simulink model "MomentumBasedController"  (R2021b)
settings: Solver=FixedStepAuto  StartTime=0.0  StopTime=Config.SIMULATION_TIME  FixedStep=Config.tStep  RelTol=1e-3
InitFcn:
  | %% initialize the simulation
  | cd(fileparts(which(bdroot)));
  | initMomentumBasedController;
StopFcn:
  | %% stop the simulation
  | cd(fileparts(which(bdroot)));
  | stopMomentumBasedController;
values from neighbouring files (symbols this model uses):
  ConfigRobot1 = ConfigRobot    [initMomentumBasedController.m]
undefined symbols (not defined in the file or in its folder): Config
libraries: RobotStateLibrary x16, WBToolboxLibrary x14, simulink x2
settings Model: Creator=lorenzorapetti  LastModifiedBy=lorenzorapetti
settings SolverCC: AlgebraicLoopSolver=TrustRegion
settings DebuggingCC: SFMachineParentedDataDiag=warning

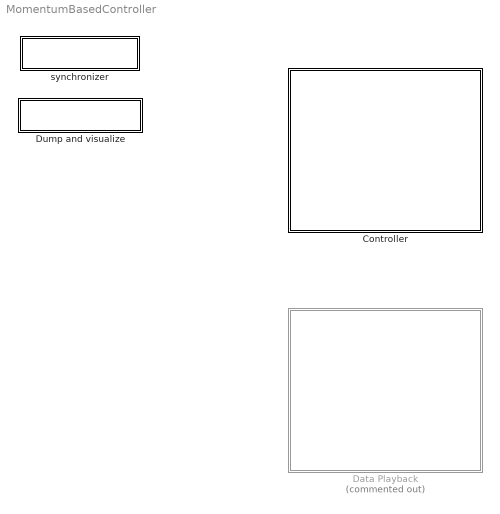
== system MomentumBasedController ==
  Controller : Subsystem
  Data Playback : Subsystem  Commented=on
  Dump and visualize : Subsystem
      mask Display: disp('VISUALIZER')
  synchronizer : Subsystem
      mask Display: disp('SYNCHRONIZER')

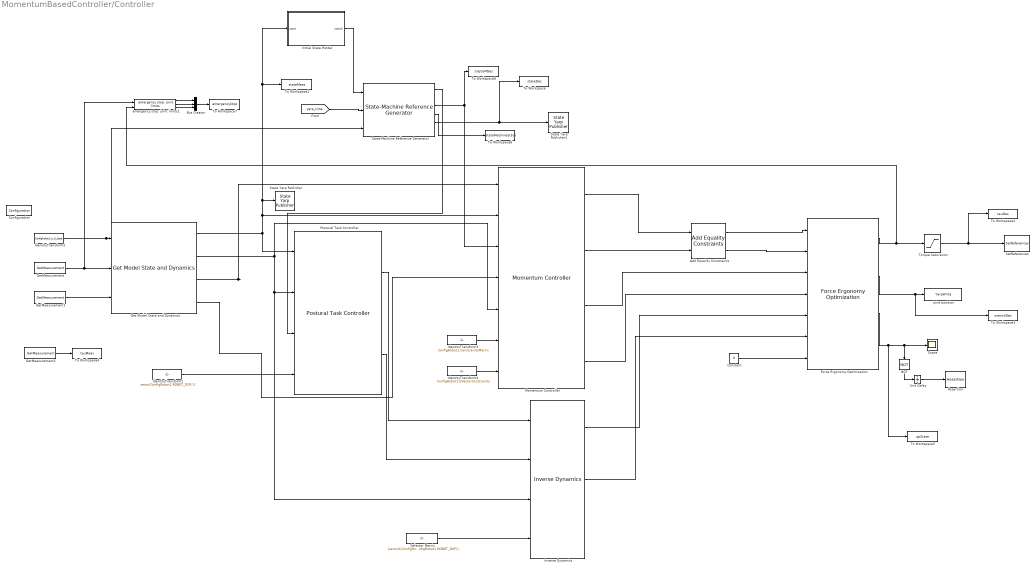
== system MomentumBasedController/Controller ==
  Add Equality Constraints : RobotStateLibrary/Add Equality Constraints  Aeq_add=ConfigRobot1.wrench_Aeq_const  beq_add=ConfigRobot1.wrench_beq_const
      settings: SourceProductName=robot-state-library
  Assertion : Assertion
  Bus Creator : BusCreator  Inputs=3
  Configuration : WBToolboxLibrary/Utilities/Configuration  ConfigSource=Workspace  ConfigObject='WBTConfigRobot_1'
      settings: SourceProductName=WholeBodyToolbox
  Constant : Constant  Value=0
  Force Ergonomy Optimization : RobotStateLibrary/Force Ergonomy Optimization  InvTol=ConfigRobot1.Reg.AInvTol  regularizationHessian=ConfigRobot1.Reg.Hessian  minimizationWeight=ConfigRobot1.Gains.tauMinimization  regularizationYDes=0
      settings: SourceProductName=robot-state-library
  Get Model State and Dynamics : RobotStateLibrary/Get Model State and Dynamics  nDoF=ConfigRobot1.ROBOT_DOF  regularization=0.001  contactFrame1Name=ConfigRobot1.Frames.LEFT_FOOT  contactFrame2Name=ConfigRobot1.Frames.RIGHT_FOOT  frame1=ConfigRobot1.Frames.LEFT_FOOT  frame2=ConfigRobot1.Frames.RIGHT_FOOT  frame3=ConfigRobot1.Frames.LEFT_HAND  frame4=ConfigRobot1.Frames.RIGHT_HAND
      settings: SourceProductName=robot-state-library
  GetMeasurement : WBToolboxLibrary/States/GetMeasurement  measuredType=Joints Position
      settings: SourceProductName=WholeBodyToolbox
  GetMeasurement1 : WBToolboxLibrary/States/GetMeasurement  measuredType=Joints Velocity
      settings: SourceProductName=WholeBodyToolbox
  GetMeasurement2 : WBToolboxLibrary/States/GetMeasurement  measuredType=Joints Torque
      settings: SourceProductName=WholeBodyToolbox
  IdentityTransform1 : Constant  Value=zeros(ConfigRobot1.ROBOT_DOF,1)
  IdentityTransform2 : Constant  Value=ConfigRobot1.w_H_base
  IdentityTransform3 : Constant  Value=ConfigRobot1.ConstraintsMatrix
  IdentityTransform4 : Constant  Value=ConfigRobot1.bVectorConstraints
  Initial State Holder : Subsystem
  Inverse Dynamics : RobotStateLibrary/Inverse Dynamics  Reg=ConfigRobot1.Reg  fixedLinkVelcityComponents=ConfigRobot1.fixedLinkVelcityComponents
      settings: SourceProductName=robot-state-library
  Momentum Controller : RobotStateLibrary/Momentum Controller  GainMomentum=ConfigRobot1.Gains.GainMomentum  linksUseConstraintMatrix=ConfigRobot1.linksUseConstraintMatrix
      settings: SourceProductName=robot-state-library
  NOT : Logic  Operator=NOT  IconShape=distinctive  AllPortsSameDT=off  OutDataTypeStr=boolean
  Postural Task Controller : RobotStateLibrary/Postural Task Controller  GainPostural=ConfigRobot1.Gains.GainPostural
      settings: SourceProductName=robot-state-library
  Scope : Scope
  Selector Matrix : Constant  Value=[zeros(6,ConfigRobot1.ROBOT_DOF); eye(ConfigRobot1.ROBOT_DOF)]
  SetReferences : WBToolboxLibrary/Actuators/SetReferences  controlType=Torque  refSpeed=10*(pi/180)  refAcceleration=1000000*(pi/180)
      settings: SourceProductName=WholeBodyToolbox
  State Yarp Publisher : RobotStateLibrary/State Yarp Publisher  basePosePortName='/collaborativeController/robot1/basePose:o'  jointPosPortName='/collaborativeController/robot1/jointPosition:o'  nuPortName='/collaborativeController/robot1/stateVelocity:o'  posCoMPortName='/collaborativeController/robot1/CoMPosition:o'
      settings: SourceProductName=robot-state-library
  State Yarp Publisher1 : RobotStateLibrary/State Yarp Publisher  basePosePortName='/collaborativeController/robotRef/basePose:o'  jointPosPortName='/collaborativeController/robotRef/jointPosition:o'  nuPortName='/collaborativeController/robotRef/stateVelocity:o'  posCoMPortName='/collaborativeController/robotRef/CoMPosition:o'
      settings: SourceProductName=robot-state-library
  State-Machine Reference Generator : RobotStateLibrary/State-Machine Reference Generator  configStateMachine=ConfigRobot1.StateMachine  sampleTime=Config.tStep  frameName1=ConfigRobot1.Frames.LEFT_FOOT  frameName2=ConfigRobot1.Frames.RIGHT_FOOT  regularization=0.001  nDoF=ConfigRobot1.ROBOT_DOF  frame1=ConfigRobot1.Frames.LEFT_FOOT  frame2=ConfigRobot1.Frames.RIGHT_FOOT  frame3=ConfigRobot1.Frames.LEFT_HAND  frame4=ConfigRobot1.Frames.RIGHT_HAND
      link override "CoM6D ->  CoMXYZ2": NumberOfDimensions=1  InputPortWidth=6
      link override "CoM6D ->  CoMXYZ5": NumberOfDimensions=1  InputPortWidth=-1
      settings: SourceProductName=robot-state-library
  To Workspace : ToWorkspace  VariableName=stateDes  SaveFormat=Timeseries  SampleTime=-1
  To Workspace1 : ToWorkspace  VariableName=stateMeas  SaveFormat=Timeseries  SampleTime=-1
  To Workspace2 : ToWorkspace  VariableName=tauDes  SaveFormat=Timeseries  SampleTime=-1
  To Workspace3 : ToWorkspace  VariableName=wrenchDes  SaveFormat=Timeseries  SampleTime=-1
  To Workspace4 : ToWorkspace  VariableName=tauMeas  SaveFormat=Timeseries  SampleTime=-1
  To Workspace5 : ToWorkspace  VariableName=qpState  SaveFormat=Timeseries  SampleTime=-1
  To Workspace6 : ToWorkspace  VariableName=stateMachineState  SaveFormat=Timeseries  SampleTime=-1
  To Workspace7 : ToWorkspace  VariableName=emergencyStop  SaveFormat=Timeseries  SampleTime=-1
  To Workspace8 : ToWorkspace  VariableName=trajCoMDes  SaveFormat=Timeseries  SampleTime=-1
  Torque Saturation : Saturate  UpperLimit=ConfigRobot1.Safety.torqueSaturation  LowerLimit=-ConfigRobot1.Safety.torqueSaturation
  Unit Delay : UnitDelay  InitialCondition=1  SampleTime=Config.tStep  HasFrameUpgradeWarning=on
  emergency stop: joint limits1 : RobotStateLibrary/emergency stop: joint limits  Safety=ConfigRobot1.Safety
      settings: SourceProductName=robot-state-library
  joint position : WBToolboxLibrary/Utilities/YarpWrite  portName='/collaborativeController/robotRef/wrench:o'  autoconnect=off  errorOnConnection=on
      settings: SourceProductName=WholeBodyToolbox
  wires:
  IdentityTransform1/1 -> Postural Task Controller/4
  GetMeasurement/1 -> emergency stop: joint limits1/1, Get Model State and Dynamics/2
  GetMeasurement1/1 -> Get Model State and Dynamics/3
  IdentityTransform2/1 -> State-Machine Reference Generator/3, Get Model State and Dynamics/1
  Get Model State and Dynamics/3 -> Momentum Controller/1
  State-Machine Reference Generator/3 -> Momentum Controller/3, To Workspace8/1
  IdentityTransform3/1 -> Momentum Controller/6
  IdentityTransform4/1 -> Momentum Controller/7
  Postural Task Controller/1 -> Inverse Dynamics/1
  Postural Task Controller/2 -> Inverse Dynamics/2
  [yarp_time] -> State-Machine Reference Generator/2
  State-Machine Reference Generator/1 -> Postural Task Controller/3
  State-Machine Reference Generator/5 -> To Workspace/1, State Yarp Publisher1/1
  Get Model State and Dynamics/1 -> Postural Task Controller/1, Momentum Controller/2, To Workspace1/1, Initial State Holder/1(state), State Yarp Publisher/1
  Initial State Holder/1(state0) -> State-Machine Reference Generator/1
  Get Model State and Dynamics/4 -> Momentum Controller/4
  Get Model State and Dynamics/2 -> Inverse Dynamics/3, Postural Task Controller/2, Momentum Controller/5
  Momentum Controller/3 -> Force Ergonomy Optimization/3
  Momentum Controller/4 -> Force Ergonomy Optimization/4
  Inverse Dynamics/1 -> Force Ergonomy Optimization/5
  Inverse Dynamics/2 -> Force Ergonomy Optimization/6
  Momentum Controller/1 -> Add Equality Constraints/1
  Add Equality Constraints/1 -> Force Ergonomy Optimization/1
  Momentum Controller/2 -> Add Equality Constraints/2
  Add Equality Constraints/2 -> Force Ergonomy Optimization/2
  Selector Matrix/1 -> Inverse Dynamics/4
  Force Ergonomy Optimization/1 -> emergency stop: joint limits1/2, Torque Saturation/1
  Torque Saturation/1 -> To Workspace2/1, SetReferences/1
  Force Ergonomy Optimization/3 -> To Workspace5/1, NOT/1, Scope/1
  Force Ergonomy Optimization/2 -> To Workspace3/1, joint position/1
  Unit Delay/1 -> Assertion/1
  NOT/1 -> Unit Delay/1
  GetMeasurement2/1 -> To Workspace4/1
  State-Machine Reference Generator/4 -> To Workspace6/1
  emergency stop: joint limits1/1 -> Bus Creator/1
  emergency stop: joint limits1/2 -> Bus Creator/2
  emergency stop: joint limits1/3 -> Bus Creator/3
  Bus Creator/1 -> To Workspace7/1
  Constant/1 -> Force Ergonomy Optimization/7

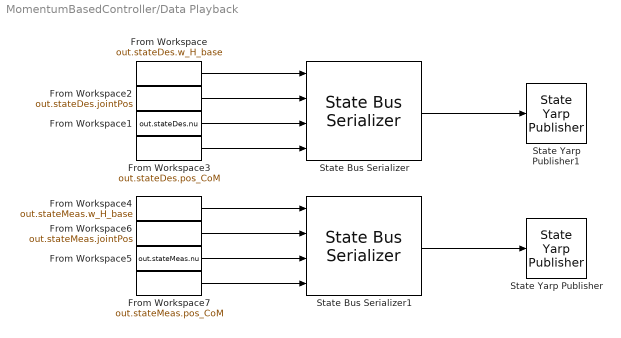
== system MomentumBasedController/Data Playback ==
  From Workspace : FromWorkspace  VariableName=out.stateDes.w_H_base  OutputAfterFinalValue=Holding final value
  From Workspace1 : FromWorkspace  VariableName=out.stateDes.nu  OutputAfterFinalValue=Holding final value
  From Workspace2 : FromWorkspace  VariableName=out.stateDes.jointPos  OutputAfterFinalValue=Holding final value
  From Workspace3 : FromWorkspace  VariableName=out.stateDes.pos_CoM  OutputAfterFinalValue=Holding final value
  From Workspace4 : FromWorkspace  VariableName=out.stateMeas.w_H_base  OutputAfterFinalValue=Holding final value
  From Workspace5 : FromWorkspace  VariableName=out.stateMeas.nu  OutputAfterFinalValue=Holding final value
  From Workspace6 : FromWorkspace  VariableName=out.stateMeas.jointPos  OutputAfterFinalValue=Holding final value
  From Workspace7 : FromWorkspace  VariableName=out.stateMeas.pos_CoM  OutputAfterFinalValue=Holding final value
  State Bus Serializer : RobotStateLibrary/State Bus Serializer  SystemSampleTime=-1  VariantActivationTime=update diagram  Latency=0  AutoFrameSizeCalculation=off
      settings: SourceProductName=robot-state-library
  State Bus Serializer1 : RobotStateLibrary/State Bus Serializer  SystemSampleTime=-1  VariantActivationTime=update diagram  Latency=0  AutoFrameSizeCalculation=off
      settings: SourceProductName=robot-state-library
  State Yarp Publisher : RobotStateLibrary/State Yarp Publisher  basePosePortName='/collaborativeController/robot1/basePose:o'  jointPosPortName='/collaborativeController/robot1/jointPosition:o'  nuPortName='/collaborativeController/robot1/stateVelocity:o'  posCoMPortName='/collaborativeController/robot1/CoMPosition:o'
      settings: SourceProductName=robot-state-library
  State Yarp Publisher1 : RobotStateLibrary/State Yarp Publisher  basePosePortName='/collaborativeController/robotRef/basePose:o'  jointPosPortName='/collaborativeController/robotRef/jointPosition:o'  nuPortName='/collaborativeController/robotRef/stateVelocity:o'  posCoMPortName='/collaborativeController/robotRef/CoMPosition:o'
      settings: SourceProductName=robot-state-library
  wires:
  From Workspace3/1 -> State Bus Serializer/4
  State Bus Serializer/1 -> State Yarp Publisher1/1
  From Workspace2/1 -> State Bus Serializer/2
  From Workspace4/1 -> State Bus Serializer1/1
  From Workspace7/1 -> State Bus Serializer1/4
  From Workspace1/1 -> State Bus Serializer/3
  From Workspace6/1 -> State Bus Serializer1/2
  State Bus Serializer1/1 -> State Yarp Publisher/1
  From Workspace5/1 -> State Bus Serializer1/3
  From Workspace/1 -> State Bus Serializer/1

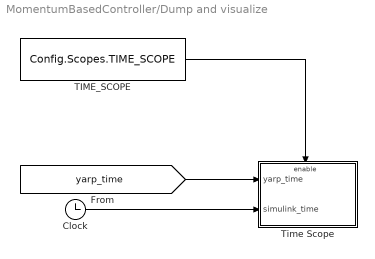
== system MomentumBasedController/Dump and visualize ==
  Clock : Clock
  TIME_SCOPE : Constant  Value=Config.Scopes.TIME_SCOPE
  Time Scope : Subsystem
  wires:
  TIME_SCOPE/1 -> Time Scope/Enable
  [yarp_time] -> Time Scope/1(yarp_time)
  Clock/1 -> Time Scope/2(simulink_time)

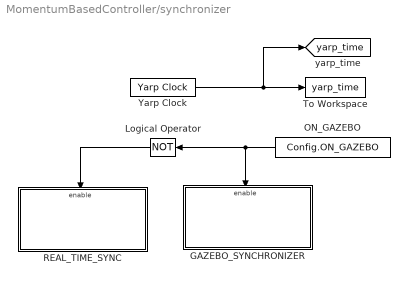
== system MomentumBasedController/synchronizer ==
  GAZEBO_SYNCHRONIZER : Subsystem
  Logical Operator : Logic  Operator=NOT  AllPortsSameDT=off  OutDataTypeStr=boolean
  "ON_GAZEBO " : Constant  Value=Config.ON_GAZEBO
  REAL_TIME_SYNC : Subsystem
  To Workspace : ToWorkspace  VariableName=yarp_time  SaveFormat=Structure With Time  SampleTime=-1
  Yarp Clock : WBToolboxLibrary/Utilities/Yarp Clock
      settings: SourceProductName=WholeBodyToolbox
  tag scope: yarp_time=global
  wires:
  Logical Operator/1 -> REAL_TIME_SYNC/Enable
  "ON_GAZEBO "/1 -> GAZEBO_SYNCHRONIZER/Enable, Logical Operator/1
  Yarp Clock/1 -> [yarp_time], To Workspace/1

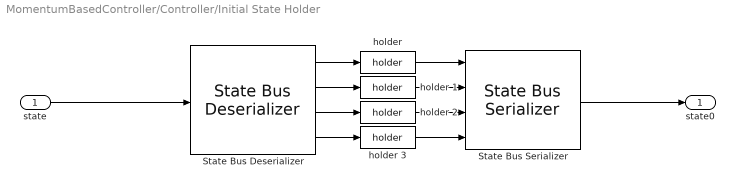
== system MomentumBasedController/Controller/Initial State Holder ==
  state : Inport
  State Bus Deserializer : RobotStateLibrary/State Bus Deserializer  SystemSampleTime=-1  VariantActivationTime=update diagram  Latency=0  AutoFrameSizeCalculation=off
      settings: SourceProductName=robot-state-library
  State Bus Serializer : RobotStateLibrary/State Bus Serializer  SystemSampleTime=-1  VariantActivationTime=update diagram  Latency=0  AutoFrameSizeCalculation=off
      settings: SourceProductName=robot-state-library
  holder {,1..3} (4 alike) : WBToolboxLibrary/Utilities/holder 
      settings: SourceProductName=WholeBodyToolbox
  state0 : Outport
  wires:
  State Bus Deserializer/2 -> holder 1/1
  State Bus Deserializer/4 -> holder 3/1
  holder 1/1 -> State Bus Serializer/2
  holder 3/1 -> State Bus Serializer/4
  State Bus Deserializer/1 -> "holder "/1
  state/1 -> State Bus Deserializer/1
  holder 2/1 -> State Bus Serializer/3
  State Bus Serializer/1 -> state0/1
  "holder "/1 -> State Bus Serializer/1
  State Bus Deserializer/3 -> holder 2/1

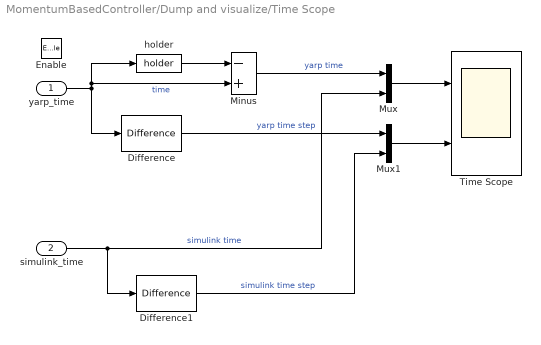
== system MomentumBasedController/Dump and visualize/Time Scope ==
  yarp_time : Inport
  simulink_time : Inport  Port=2
  Enable : EnablePort
  Difference : simulink/Discrete/Difference  ICPrevInput=0.0  OutMin=[]  OutMax=[]  OutDataType=fixdt(1, 16)  OutScaling=2^-10  DoSatur=off
  Difference1 : simulink/Discrete/Difference  ICPrevInput=0.0  OutMin=[]  OutMax=[]  OutDataType=fixdt(1, 16)  OutScaling=2^-10  DoSatur=off
  Minus : Sum  Inputs=-+
  Mux : Mux  Inputs=2
  Mux1 : Mux  Inputs=2
  Time Scope : Scope  NumInputPorts=2
  "holder " : WBToolboxLibrary/Utilities/holder 
      settings: SourceProductName=WholeBodyToolbox
  wires:
  yarp_time/1 -> "holder "/1, Minus/2, Difference/1  "time"
  "holder "/1 -> Minus/1
  simulink_time/1 -> Mux/2, Difference1/1  "simulink time"
  Minus/1 -> Mux/1  "yarp time"
  Mux/1 -> Time Scope/1
  Difference/1 -> Mux1/1  "yarp time step"
  Difference1/1 -> Mux1/2  "simulink time step"
  Mux1/1 -> Time Scope/2

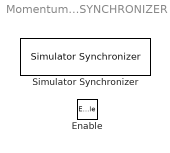
== system MomentumBasedController/synchronizer/GAZEBO_SYNCHRONIZER ==
  Enable : EnablePort
  Simulator Synchronizer : WBToolboxLibrary/Utilities/Simulator Synchronizer  period=Config.tStep  serverPortName='/clock/rpc'  clientPortName='/WBT_synchronizer/rpc:o'
      settings: SourceProductName=WholeBodyToolbox

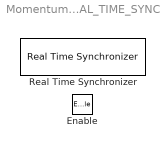
== system MomentumBasedController/synchronizer/REAL_TIME_SYNC ==
  Enable : EnablePort
  Real Time Synchronizer : WBToolboxLibrary/Utilities/Real Time Synchronizer  period=Config.tStep
      settings: SourceProductName=WholeBodyToolbox
